simulink model "CombineHandAutomatic"  (R2015b)
settings: Solver=ode1  StartTime=0.0  StopTime=180  FixedStep=0.1  RelTol=1e-3
settings Model: Creator=METZLER  LastModifiedBy=METZLER

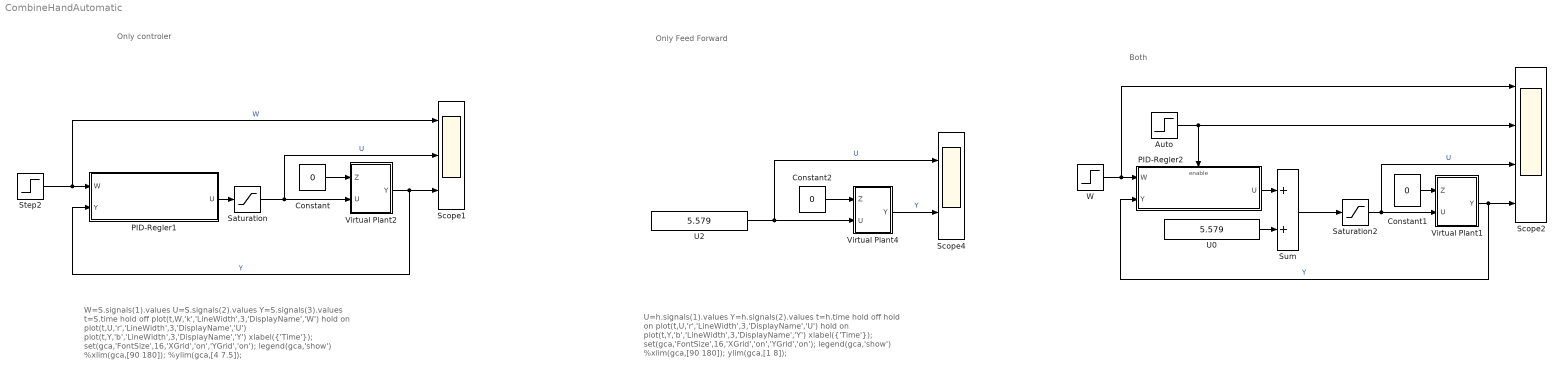
== system CombineHandAutomatic ==
  note: Both
  note: Only Feed Forward
  note: Only controler
  note: W=S.signals(1).values
      | U=S.signals(2).values
      | Y=S.signals(3).values
      | t=S.time
      | hold off
      | plot(t,W,'k','LineWidth',3,'DisplayName','W')
      | hold on
      | plot(t,U,'r','LineWidth',3,'DisplayName','U')
      | plot(t,Y,'b','LineWidth',3,'DisplayName','Y')
      | xlabel({'Time'});
      | set(gca,'FontSize',16,'XGrid','on','YGrid','on');
      | legend(gca,'show')
      | %xlim(gca,[90 180]);
      | %ylim(gca,[4 7.5]);
  note: U=h.signals(1).values
      | Y=h.signals(2).values
      | t=h.time
      | hold off
      | hold on
      | plot(t,U,'r','LineWidth',3,'DisplayName','U')
      | hold on
      | plot(t,Y,'b','LineWidth',3,'DisplayName','Y')
      | xlabel({'Time'});
      | set(gca,'FontSize',16,'XGrid','on','YGrid','on');
      | legend(gca,'show')
      | %xlim(gca,[90 180]);
      | ylim(gca,[1 8]);
  Auto : Step  Time=30  SampleTime=0
  Constant : Constant  Value=0
  Constant1 : Constant  Value=0
  Constant2 : Constant  Value=0
  PID-Regler1 : Subsystem  mask{cpc=0.7702, cic=0.1621, cdc=0.8783, T=0.1}
      mask prompts: T "T  Time constant of real D-Part"
      mask help: A simple PID-Controller for the MOOC MSUS
      mask Display:
      | IconText='';
      | if ~strcmp(get_param(gcb,'cpc'),'0')
      |     IconText=strcat(IconText,'P');
      | end
      | if ~strcmp(get_param(gcb,'cic'),'0')
      |    IconText=strcat(IconText,'I');
      | end
      | if ~strcmp(get_param(gcb,'cdc'),'0')
      |     IconText=strcat(IconText,'D');
      | end
      | IconText=strcat(IconText,'-Controller')
      | plot(0,0)
      | plot(100,100)
      | text(25,50,IconText)
      | port_label ('output',1,'U')
      | port_label ('input',1,'W')
      | port_label ('input',2,'Y')
  PID-Regler2 : Subsystem  mask{cpc=0.7702, cic=0.1621, cdc=0.8783, T=0.1}
      mask prompts: T "T  Time constant of real D-Part"
      mask help: A simple PID-Controller for the MOOC MSUS
      mask Display:
      | IconText='';
      | if ~strcmp(get_param(gcb,'cpc'),'0')
      |     IconText=strcat(IconText,'P');
      | end
      | if ~strcmp(get_param(gcb,'cic'),'0')
      |    IconText=strcat(IconText,'I');
      | end
      | if ~strcmp(get_param(gcb,'cdc'),'0')
      |     IconText=strcat(IconText,'D');
      | end
      | IconText=strcat(IconText,'-Controller')
      | plot(0,0)
      | plot(100,100)
      | text(25,50,IconText)
      | port_label ('output',1,'U')
      | port_label ('input',1,'W')
      | port_label ('input',2,'Y')
  Saturation : Saturate  UpperLimit=7.5  LowerLimit=4.5
      settings: AttributesFormatString=|
      | Lower Limit=%<LowerLimit>
      | Upper Limit=%<UpperLimit>
  Saturation2 : Saturate  UpperLimit=7.5  LowerLimit=4.5
      settings: AttributesFormatString=|
      | Lower Limit=%<LowerLimit>
      | Upper Limit=%<UpperLimit>
  Scope1 : Scope  NumInputPorts=3
  Scope2 : Scope  NumInputPorts=4
  Scope4 : Scope  NumInputPorts=2
  Step2 : Step  Time=100  Before=4  After=6  SampleTime=0
      settings: AttributesFormatString=|
      | Start Value=%<Before>
      | Step Time=%<Time>
      | Final Vlaue=%<After>
  Sum : Sum
  U0 : Constant  Value=5.579  OutDataTypeStr=double
  U2 : Constant  Value=5.579  OutDataTypeStr=double
  Virtual Plant1 : Subsystem
  Virtual Plant2 : Subsystem
  Virtual Plant4 : Subsystem
  W : Step  Time=100  Before=4  After=6  SampleTime=0
  wires:
  PID-Regler1/1(U) -> Saturation/1
  Step2/1 -> PID-Regler1/1(W), Scope1/1  "W"
  Virtual Plant2/1(Y) -> Scope1/3, PID-Regler1/2(Y)  "Y"
  Constant/1 -> Virtual Plant2/1(Z)
  Saturation/1 -> Virtual Plant2/2(U), Scope1/2  "U"
  PID-Regler2/1(U) -> Sum/1
  Virtual Plant1/1(Y) -> Scope2/4, PID-Regler2/2(Y)  "Y"
  Constant1/1 -> Virtual Plant1/1(Z)
  Saturation2/1 -> Virtual Plant1/2(U), Scope2/3  "U"
  U0/1 -> Sum/2
  Sum/1 -> Saturation2/1
  Auto/1 -> PID-Regler2/Enable, Scope2/2
  W/1 -> Scope2/1, PID-Regler2/1(W)
  Constant2/1 -> Virtual Plant4/1(Z)
  U2/1 -> Scope4/1, Virtual Plant4/2(U)  "U"
  Virtual Plant4/1(Y) -> Scope4/2  "Y"

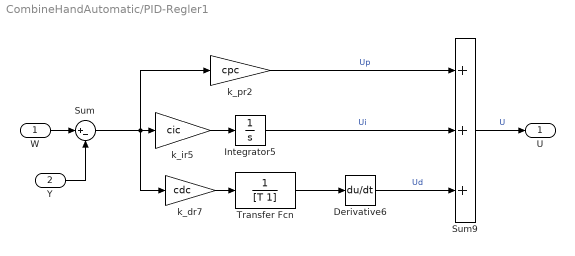
== system CombineHandAutomatic/PID-Regler1 ==
  W : Inport
  Y : Inport  Port=2
  Derivative6 : Derivative
  Integrator5 : Integrator
  Sum : Sum  Inputs=|+-
  Sum9 : Sum  Inputs=+++
  Transfer Fcn : TransferFcn  Denominator=[T 1]
  k_dr7 : Gain  Gain=cdc
  k_ir5 : Gain  Gain=cic
  k_pr2 : Gain  Gain=cpc
  U : Outport
  wires:
  Y/1 -> Sum/2
  Sum9/1 -> U/1  "U"
  W/1 -> Sum/1
  Derivative6/1 -> Sum9/3  "Ud"
  k_pr2/1 -> Sum9/1  "Up"
  k_ir5/1 -> Integrator5/1
  Integrator5/1 -> Sum9/2  "Ui"
  Transfer Fcn/1 -> Derivative6/1
  k_dr7/1 -> Transfer Fcn/1
  Sum/1 -> k_ir5/1, k_pr2/1, k_dr7/1

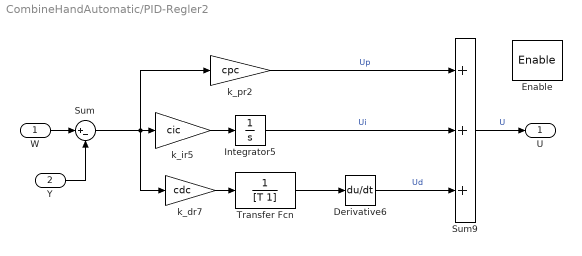
== system CombineHandAutomatic/PID-Regler2 ==
  W : Inport
  Y : Inport  Port=2
  Enable : EnablePort
  Derivative6 : Derivative
  Integrator5 : Integrator
  Sum : Sum  Inputs=|+-
  Sum9 : Sum  Inputs=+++
  Transfer Fcn : TransferFcn  Denominator=[T 1]
  k_dr7 : Gain  Gain=cdc
  k_ir5 : Gain  Gain=cic
  k_pr2 : Gain  Gain=cpc
  U : Outport
  wires:
  Y/1 -> Sum/2
  Sum9/1 -> U/1  "U"
  W/1 -> Sum/1
  Derivative6/1 -> Sum9/3  "Ud"
  k_pr2/1 -> Sum9/1  "Up"
  k_ir5/1 -> Integrator5/1
  Integrator5/1 -> Sum9/2  "Ui"
  Transfer Fcn/1 -> Derivative6/1
  k_dr7/1 -> Transfer Fcn/1
  Sum/1 -> k_ir5/1, k_pr2/1, k_dr7/1

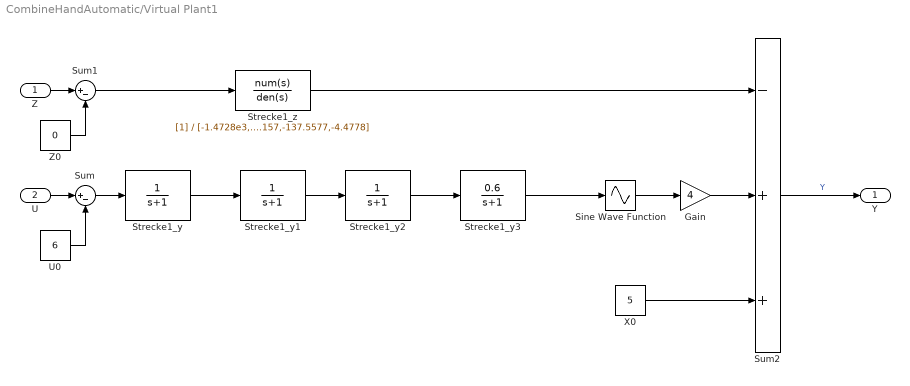
== system CombineHandAutomatic/Virtual Plant1 ==
  Z : Inport
  U : Inport  Port=2
  Gain : Gain  Gain=4
  Sine Wave Function : Sin  TimeSource=Use external signal  SampleTime=0
  Strecke1_y : TransferFcn  Denominator=[1,1]
  Strecke1_y1 : TransferFcn  Denominator=[1,1]
  Strecke1_y2 : TransferFcn  Denominator=[1,1]
  Strecke1_y3 : TransferFcn  Numerator=[0.6]  Denominator=[1,1]
  Strecke1_z : TransferFcn  Denominator=[-1.4728e3,-534.157,-137.5577,-4.4778]
  Sum : Sum  Inputs=|+-
  Sum1 : Sum  Inputs=|+-
  Sum2 : Sum  Inputs=-++
  U0 : Constant  Value=6
  X0 : Constant  Value=5
  Z0 : Constant  Value=0
  Y : Outport
  wires:
  Sum2/1 -> Y/1  "Y"
  U/1 -> Sum/1
  Z/1 -> Sum1/1
  X0/1 -> Sum2/3
  Strecke1_z/1 -> Sum2/1
  Z0/1 -> Sum1/2
  Sum1/1 -> Strecke1_z/1
  U0/1 -> Sum/2
  Sum/1 -> Strecke1_y/1
  Strecke1_y/1 -> Strecke1_y1/1
  Strecke1_y1/1 -> Strecke1_y2/1
  Strecke1_y2/1 -> Strecke1_y3/1
  Strecke1_y3/1 -> Sine Wave Function/1
  Sine Wave Function/1 -> Gain/1
  Gain/1 -> Sum2/2

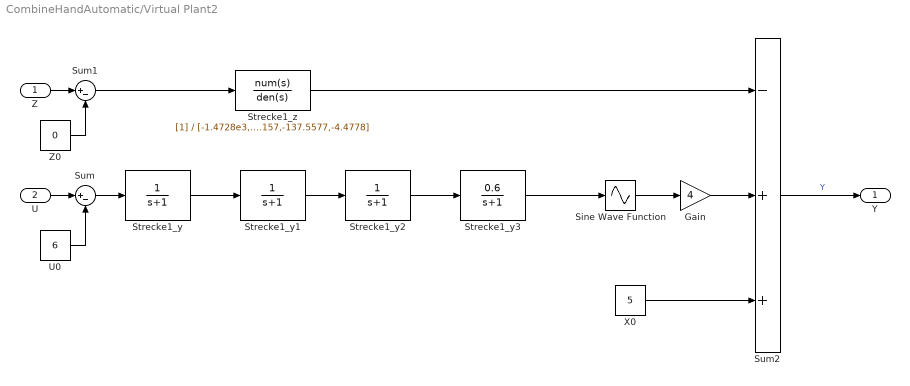
== system CombineHandAutomatic/Virtual Plant2 ==
  Z : Inport
  U : Inport  Port=2
  Gain : Gain  Gain=4
  Sine Wave Function : Sin  TimeSource=Use external signal  SampleTime=0
  Strecke1_y : TransferFcn  Denominator=[1,1]
  Strecke1_y1 : TransferFcn  Denominator=[1,1]
  Strecke1_y2 : TransferFcn  Denominator=[1,1]
  Strecke1_y3 : TransferFcn  Numerator=[0.6]  Denominator=[1,1]
  Strecke1_z : TransferFcn  Denominator=[-1.4728e3,-534.157,-137.5577,-4.4778]
  Sum : Sum  Inputs=|+-
  Sum1 : Sum  Inputs=|+-
  Sum2 : Sum  Inputs=-++
  U0 : Constant  Value=6
  X0 : Constant  Value=5
  Z0 : Constant  Value=0
  Y : Outport
  wires:
  Sum2/1 -> Y/1  "Y"
  U/1 -> Sum/1
  Z/1 -> Sum1/1
  X0/1 -> Sum2/3
  Strecke1_z/1 -> Sum2/1
  Z0/1 -> Sum1/2
  Sum1/1 -> Strecke1_z/1
  U0/1 -> Sum/2
  Sum/1 -> Strecke1_y/1
  Strecke1_y/1 -> Strecke1_y1/1
  Strecke1_y1/1 -> Strecke1_y2/1
  Strecke1_y2/1 -> Strecke1_y3/1
  Strecke1_y3/1 -> Sine Wave Function/1
  Sine Wave Function/1 -> Gain/1
  Gain/1 -> Sum2/2

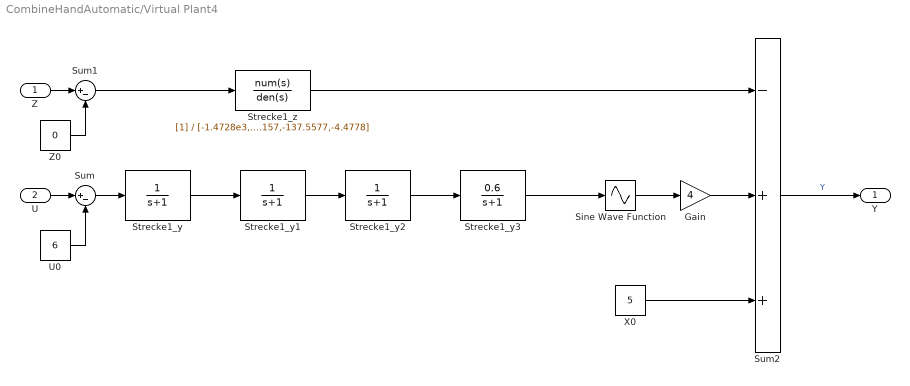
== system CombineHandAutomatic/Virtual Plant4 ==
  Z : Inport
  U : Inport  Port=2
  Gain : Gain  Gain=4
  Sine Wave Function : Sin  TimeSource=Use external signal  SampleTime=0
  Strecke1_y : TransferFcn  Denominator=[1,1]
  Strecke1_y1 : TransferFcn  Denominator=[1,1]
  Strecke1_y2 : TransferFcn  Denominator=[1,1]
  Strecke1_y3 : TransferFcn  Numerator=[0.6]  Denominator=[1,1]
  Strecke1_z : TransferFcn  Denominator=[-1.4728e3,-534.157,-137.5577,-4.4778]
  Sum : Sum  Inputs=|+-
  Sum1 : Sum  Inputs=|+-
  Sum2 : Sum  Inputs=-++
  U0 : Constant  Value=6
  X0 : Constant  Value=5
  Z0 : Constant  Value=0
  Y : Outport
  wires:
  Sum2/1 -> Y/1  "Y"
  U/1 -> Sum/1
  Z/1 -> Sum1/1
  X0/1 -> Sum2/3
  Strecke1_z/1 -> Sum2/1
  Z0/1 -> Sum1/2
  Sum1/1 -> Strecke1_z/1
  U0/1 -> Sum/2
  Sum/1 -> Strecke1_y/1
  Strecke1_y/1 -> Strecke1_y1/1
  Strecke1_y1/1 -> Strecke1_y2/1
  Strecke1_y2/1 -> Strecke1_y3/1
  Strecke1_y3/1 -> Sine Wave Function/1
  Sine Wave Function/1 -> Gain/1
  Gain/1 -> Sum2/2
